simulink model "pwm_deadtime_compensation_model"  (R2023b)
settings: Solver=FixedStepDiscrete  StartTime=0.0  StopTime=deadtime_comp_defaults.simcfg.stop_time  FixedStep=deadtime_comp_defaults.simcfg.Ts_step  RelTol=1e-3
values from neighbouring files (symbols this model uses):
  DeadtimeCompCurrentInvRange_1perA = 12.5    [pwm_deadtime_compensation_interface.sldd]
  DeadtimeCompCurrentZero_A = 0.019999999552965164    [pwm_deadtime_compensation_interface.sldd]
  DeadtimeCompDuty = 0.0099999997764825821    [pwm_deadtime_compensation_interface.sldd]
  DeadtimeCompEnable = 1.0    [pwm_deadtime_compensation_interface.sldd]
  DeadtimeCompPolarity = -1.0    [pwm_deadtime_compensation_interface.sldd]
undefined symbols (not defined in the file or in its folder): deadtime_comp_defaults, deadtime_comp_test
settings Model: DataDictionary=pwm_deadtime_compensation_interface.sldd  Creator=user  LastModifiedBy=user
settings OptimizationCC: DefaultParameterBehavior=Inlined  EnhancedBackFolding=on  PassReuseOutputArgsAs=Individual arguments  OptimizeBlockOrder=speed  DifferentSizesBufferReuse=on  OptimizationCustomize=off  EfficientTunableParamExpr=on
settings DebuggingCC: ParameterTunabilityLossMsg=error
settings HardwareCC: ProdBitPerPointer=32  ProdBitPerSizeT=32  ProdBitPerPtrDiffT=32  ProdLargestAtomicInteger=Long  ProdLargestAtomicFloat=Double  ProdWordSize=32  ProdHWDeviceType=ARM Compatible->ARM Cortex  TargetLargestAtomicInteger=Long  TargetLargestAtomicFloat=Double  TargetIntDivRoundTo=Zero  TargetEndianess=LittleEndian  TargetHWDeviceType=ARM Compatible->ARM Cortex  ProdEqTarget=off
settings SFSimCC: MATLABDynamicMemAlloc=off
settings RTWCC: Description=Embedded Coder  SystemTargetFile=ert.tlc  GenCodeOnly=on  TemplateMakefile=ert_default_tmf  GenerateReport=on
settings CodeAppCC: ForceParamTrailComments=on  IgnoreCustomStorageClasses=off  OperatorAnnotations=on  SimulinkDataObjDesc=on  SFDataObjDesc=on  InsertBlockDesc=on
settings ERTTargetCC: TargetLangStandard=C99 (ISO)  CodeInterfacePackaging=Reusable function  InlinedParameterPlacement=NonHierarchical  ERTCustomFileTemplate=example_file_process.tlc

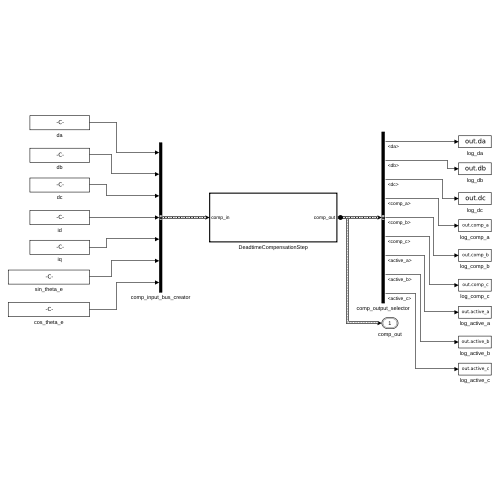
[thumbnail: Simulink's stored preview of the top-level diagram]
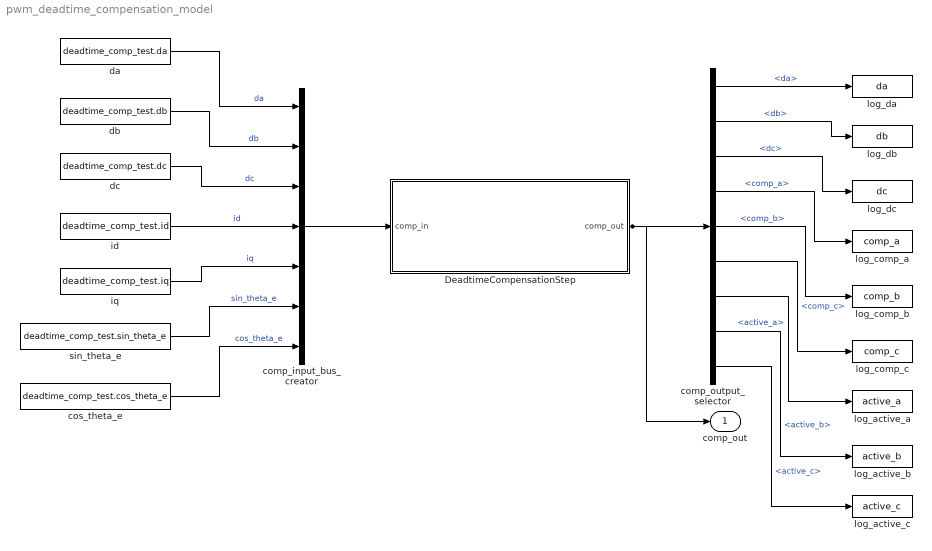
== system pwm_deadtime_compensation_model ==
  DeadtimeCompensationStep : Subsystem  TreatAsAtomicUnit=on  RTWFcnName=DeadtimeCompensationStep  RTWFileName=DeadtimeCompensationStep
      settings: RTWFcnNameOpts=User specified  RTWFileNameOpts=User specified
  comp_input_bus_creator : BusCreator  Inputs=7  OutDataTypeStr=Bus: pwm_deadtime_comp_input_t  NonVirtualBus=on
  comp_output_selector : BusSelector  OutputSignals=da,db,dc,comp_a,comp_b,comp_c,active_a,active_b,active_c
  cos_theta_e : Constant  Value=deadtime_comp_test.cos_theta_e  OutDataTypeStr=T_DeadtimeCompTrig  SampleTime=deadtime_comp_defaults.simcfg.Ts_step
  da : Constant  Value=deadtime_comp_test.da  OutDataTypeStr=T_DeadtimeCompDuty  SampleTime=deadtime_comp_defaults.simcfg.Ts_step
  db : Constant  Value=deadtime_comp_test.db  OutDataTypeStr=T_DeadtimeCompDuty  SampleTime=deadtime_comp_defaults.simcfg.Ts_step
  dc : Constant  Value=deadtime_comp_test.dc  OutDataTypeStr=T_DeadtimeCompDuty  SampleTime=deadtime_comp_defaults.simcfg.Ts_step
  id : Constant  Value=deadtime_comp_test.id  OutDataTypeStr=T_DeadtimeCompCurrent  SampleTime=deadtime_comp_defaults.simcfg.Ts_step
  iq : Constant  Value=deadtime_comp_test.iq  OutDataTypeStr=T_DeadtimeCompCurrent  SampleTime=deadtime_comp_defaults.simcfg.Ts_step
  log_active_a : ToWorkspace  VariableName=active_a  SaveFormat=Structure With Time  SampleTime=-1
  log_active_b : ToWorkspace  VariableName=active_b  SaveFormat=Structure With Time  SampleTime=-1
  log_active_c : ToWorkspace  VariableName=active_c  SaveFormat=Structure With Time  SampleTime=-1
  log_comp_a : ToWorkspace  VariableName=comp_a  SaveFormat=Structure With Time  SampleTime=-1
  log_comp_b : ToWorkspace  VariableName=comp_b  SaveFormat=Structure With Time  SampleTime=-1
  log_comp_c : ToWorkspace  VariableName=comp_c  SaveFormat=Structure With Time  SampleTime=-1
  log_da : ToWorkspace  VariableName=da  SaveFormat=Structure With Time  SampleTime=-1
  log_db : ToWorkspace  VariableName=db  SaveFormat=Structure With Time  SampleTime=-1
  log_dc : ToWorkspace  VariableName=dc  SaveFormat=Structure With Time  SampleTime=-1
  sin_theta_e : Constant  Value=deadtime_comp_test.sin_theta_e  OutDataTypeStr=T_DeadtimeCompTrig  SampleTime=deadtime_comp_defaults.simcfg.Ts_step
  comp_out : Outport  OutDataTypeStr=Bus: pwm_deadtime_comp_output_t  PortDimensions=1
  wires:
  comp_output_selector/7 -> log_active_a/1  "<active_a>"
  comp_output_selector/6 -> log_comp_c/1  "<comp_c>"
  da/1 -> comp_input_bus_creator/1  "da"
  dc/1 -> comp_input_bus_creator/3  "dc"
  db/1 -> comp_input_bus_creator/2  "db"
  DeadtimeCompensationStep/1(comp_out) -> comp_output_selector/1, comp_out/1
  id/1 -> comp_input_bus_creator/4  "id"
  iq/1 -> comp_input_bus_creator/5  "iq"
  sin_theta_e/1 -> comp_input_bus_creator/6  "sin_theta_e"
  comp_output_selector/5 -> log_comp_b/1  "<comp_b>"
  cos_theta_e/1 -> comp_input_bus_creator/7  "cos_theta_e"
  comp_output_selector/8 -> log_active_b/1  "<active_b>"
  comp_input_bus_creator/1 -> DeadtimeCompensationStep/1(comp_in)
  comp_output_selector/9 -> log_active_c/1  "<active_c>"
  comp_output_selector/2 -> log_db/1  "<db>"
  comp_output_selector/3 -> log_dc/1  "<dc>"
  comp_output_selector/1 -> log_da/1  "<da>"
  comp_output_selector/4 -> log_comp_a/1  "<comp_a>"

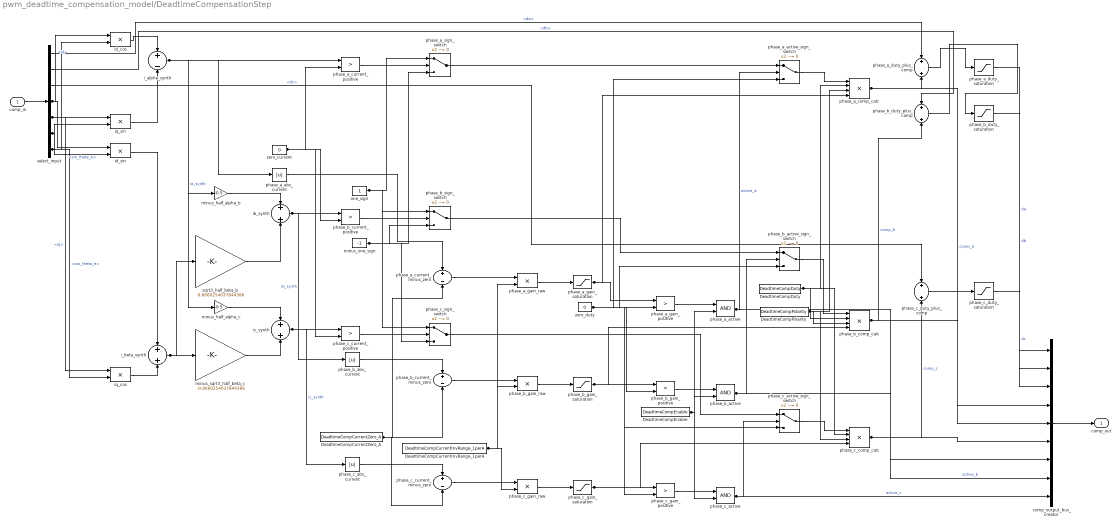
== system pwm_deadtime_compensation_model/DeadtimeCompensationStep ==
  comp_in : Inport  OutDataTypeStr=Bus: pwm_deadtime_comp_input_t  PortDimensions=1  BusOutputAsStruct=on
  DeadtimeCompCurrentInvRange_1perA : Constant  Value=DeadtimeCompCurrentInvRange_1perA  OutDataTypeStr=T_DeadtimeCompDuty  SampleTime=-1
  DeadtimeCompCurrentZero_A : Constant  Value=DeadtimeCompCurrentZero_A  OutDataTypeStr=T_DeadtimeCompCurrent  SampleTime=-1
  DeadtimeCompDuty : Constant  Value=DeadtimeCompDuty  OutDataTypeStr=T_DeadtimeCompDuty  SampleTime=-1
  DeadtimeCompEnable : Constant  Value=DeadtimeCompEnable  OutDataTypeStr=T_DeadtimeCompBool  SampleTime=-1
  DeadtimeCompPolarity : Constant  Value=DeadtimeCompPolarity  OutDataTypeStr=T_DeadtimeCompDuty  SampleTime=-1
  comp_output_bus_creator : BusCreator  Inputs=9  OutDataTypeStr=Bus: pwm_deadtime_comp_output_t  NonVirtualBus=on
  i_alpha_synth : Sum  Inputs=+-  OutDataTypeStr=T_DeadtimeCompCurrent
  i_beta_synth : Sum  OutDataTypeStr=T_DeadtimeCompCurrent
  ib_synth : Sum  OutDataTypeStr=T_DeadtimeCompCurrent
  ic_synth : Sum  OutDataTypeStr=T_DeadtimeCompCurrent
  id_cos : Product  Inputs=**  OutDataTypeStr=T_DeadtimeCompCurrent
  id_sin : Product  Inputs=**  OutDataTypeStr=T_DeadtimeCompCurrent
  iq_cos : Product  Inputs=**  OutDataTypeStr=T_DeadtimeCompCurrent
  iq_sin : Product  Inputs=**  OutDataTypeStr=T_DeadtimeCompCurrent
  minus_half_alpha_b : Gain  Gain=-0.5  OutDataTypeStr=T_DeadtimeCompCurrent
  minus_half_alpha_c : Gain  Gain=-0.5  OutDataTypeStr=T_DeadtimeCompCurrent
  minus_one_sign : Constant  Value=-1  OutDataTypeStr=T_DeadtimeCompDuty  SampleTime=-1
  minus_sqrt3_half_beta_c : Gain  Gain=-0.8660254037844386  OutDataTypeStr=T_DeadtimeCompCurrent
  one_sign : Constant  OutDataTypeStr=T_DeadtimeCompDuty  SampleTime=-1
  phase_a_abs_current : Abs  SaturateOnIntegerOverflow=off
  phase_a_active : Logic  AllPortsSameDT=off  OutDataTypeStr=T_DeadtimeCompBool
  phase_a_active_sign_switch : Switch  Criteria=u2 ~= 0  OutDataTypeStr=T_DeadtimeCompDuty  SaturateOnIntegerOverflow=off  InputSameDT=off
  phase_a_comp_calc : Product  Inputs=****  OutDataTypeStr=T_DeadtimeCompDuty
  phase_a_current_minus_zero : Sum  Inputs=+-  OutDataTypeStr=T_DeadtimeCompCurrent
  phase_a_current_positive : RelationalOperator  Operator=>  OutDataTypeStr=boolean  RndMeth=Simplest  InputSameDT=off
  phase_a_duty_plus_comp : Sum  OutDataTypeStr=T_DeadtimeCompDuty
  phase_a_duty_saturation : Saturate  UpperLimit=1  LowerLimit=0  OutDataTypeStr=T_DeadtimeCompDuty
  phase_a_gain_positive : RelationalOperator  Operator=>  OutDataTypeStr=boolean  RndMeth=Simplest  InputSameDT=off
  phase_a_gain_raw : Product  Inputs=**  OutDataTypeStr=T_DeadtimeCompDuty
  phase_a_gain_saturation : Saturate  UpperLimit=1  LowerLimit=0  OutDataTypeStr=T_DeadtimeCompDuty
  phase_a_sign_switch : Switch  Criteria=u2 ~= 0  OutDataTypeStr=T_DeadtimeCompDuty  SaturateOnIntegerOverflow=off  InputSameDT=off
  phase_b_abs_current : Abs  SaturateOnIntegerOverflow=off
  phase_b_active : Logic  AllPortsSameDT=off  OutDataTypeStr=T_DeadtimeCompBool
  phase_b_active_sign_switch : Switch  Criteria=u2 ~= 0  OutDataTypeStr=T_DeadtimeCompDuty  SaturateOnIntegerOverflow=off  InputSameDT=off
  phase_b_comp_calc : Product  Inputs=****  OutDataTypeStr=T_DeadtimeCompDuty
  phase_b_current_minus_zero : Sum  Inputs=+-  OutDataTypeStr=T_DeadtimeCompCurrent
  phase_b_current_positive : RelationalOperator  Operator=>  OutDataTypeStr=boolean  RndMeth=Simplest  InputSameDT=off
  phase_b_duty_plus_comp : Sum  OutDataTypeStr=T_DeadtimeCompDuty
  phase_b_duty_saturation : Saturate  UpperLimit=1  LowerLimit=0  OutDataTypeStr=T_DeadtimeCompDuty
  phase_b_gain_positive : RelationalOperator  Operator=>  OutDataTypeStr=boolean  RndMeth=Simplest  InputSameDT=off
  phase_b_gain_raw : Product  Inputs=**  OutDataTypeStr=T_DeadtimeCompDuty
  phase_b_gain_saturation : Saturate  UpperLimit=1  LowerLimit=0  OutDataTypeStr=T_DeadtimeCompDuty
  phase_b_sign_switch : Switch  Criteria=u2 ~= 0  OutDataTypeStr=T_DeadtimeCompDuty  SaturateOnIntegerOverflow=off  InputSameDT=off
  phase_c_abs_current : Abs  SaturateOnIntegerOverflow=off
  phase_c_active : Logic  AllPortsSameDT=off  OutDataTypeStr=T_DeadtimeCompBool
  phase_c_active_sign_switch : Switch  Criteria=u2 ~= 0  OutDataTypeStr=T_DeadtimeCompDuty  SaturateOnIntegerOverflow=off  InputSameDT=off
  phase_c_comp_calc : Product  Inputs=****  OutDataTypeStr=T_DeadtimeCompDuty
  phase_c_current_minus_zero : Sum  Inputs=+-  OutDataTypeStr=T_DeadtimeCompCurrent
  phase_c_current_positive : RelationalOperator  Operator=>  OutDataTypeStr=boolean  RndMeth=Simplest  InputSameDT=off
  phase_c_duty_plus_comp : Sum  OutDataTypeStr=T_DeadtimeCompDuty
  phase_c_duty_saturation : Saturate  UpperLimit=1  LowerLimit=0  OutDataTypeStr=T_DeadtimeCompDuty
  phase_c_gain_positive : RelationalOperator  Operator=>  OutDataTypeStr=boolean  RndMeth=Simplest  InputSameDT=off
  phase_c_gain_raw : Product  Inputs=**  OutDataTypeStr=T_DeadtimeCompDuty
  phase_c_gain_saturation : Saturate  UpperLimit=1  LowerLimit=0  OutDataTypeStr=T_DeadtimeCompDuty
  phase_c_sign_switch : Switch  Criteria=u2 ~= 0  OutDataTypeStr=T_DeadtimeCompDuty  SaturateOnIntegerOverflow=off  InputSameDT=off
  select_input : BusSelector  OutputSignals=da,db,dc,id,iq,sin_theta_e,cos_theta_e
  sqrt3_half_beta_b : Gain  Gain=0.8660254037844386  OutDataTypeStr=T_DeadtimeCompCurrent
  zero_current : Constant  Value=0  OutDataTypeStr=T_DeadtimeCompCurrent  SampleTime=-1
  zero_duty : Constant  Value=0  OutDataTypeStr=T_DeadtimeCompDuty  SampleTime=-1
  comp_out : Outport  OutDataTypeStr=Bus: pwm_deadtime_comp_output_t  PortDimensions=1
  wires:
  comp_output_bus_creator/1 -> comp_out/1
  phase_b_duty_saturation/1 -> comp_output_bus_creator/2  "db"
  phase_a_duty_saturation/1 -> comp_output_bus_creator/1  "da"
  phase_b_duty_plus_comp/1 -> phase_b_duty_saturation/1
  phase_a_duty_plus_comp/1 -> phase_a_duty_saturation/1
  DeadtimeCompCurrentZero_A/1 -> phase_a_current_minus_zero/2, phase_b_current_minus_zero/2, phase_c_current_minus_zero/2
  ib_synth/1 -> phase_b_current_positive/1, phase_b_abs_current/1  "ib_synth"
  phase_a_current_positive/1 -> phase_a_sign_switch/2
  phase_c_current_positive/1 -> phase_c_sign_switch/2
  phase_b_current_positive/1 -> phase_b_sign_switch/2
  select_input/2 -> phase_b_duty_plus_comp/1  "<db>"
  minus_half_alpha_c/1 -> ic_synth/1
  sqrt3_half_beta_b/1 -> ib_synth/2
  one_sign/1 -> phase_b_sign_switch/1, phase_a_sign_switch/1, phase_c_sign_switch/1
  phase_a_current_minus_zero/1 -> phase_a_gain_raw/1
  phase_b_gain_positive/1 -> phase_b_active/1
  minus_one_sign/1 -> phase_b_sign_switch/3, phase_c_sign_switch/3, phase_a_sign_switch/3
  phase_c_duty_saturation/1 -> comp_output_bus_creator/3  "dc"
  select_input/5 -> iq_cos/1, iq_sin/1  "<iq>"
  ic_synth/1 -> phase_c_current_positive/1, phase_c_abs_current/1  "ic_synth"
  phase_a_abs_current/1 -> phase_a_current_minus_zero/1
  phase_c_gain_saturation/1 -> phase_c_gain_positive/1, phase_c_comp_calc/4
  i_beta_synth/1 -> minus_sqrt3_half_beta_c/1, sqrt3_half_beta_b/1
  iq_sin/1 -> i_alpha_synth/2
  DeadtimeCompDuty/1 -> phase_b_comp_calc/2, phase_c_comp_calc/2, phase_a_comp_calc/2
  select_input/3 -> phase_c_duty_plus_comp/1  "<dc>"
  phase_b_abs_current/1 -> phase_b_current_minus_zero/1
  DeadtimeCompEnable/1 -> phase_b_active/2, phase_c_active/2, phase_a_active/2
  iq_cos/1 -> i_beta_synth/2
  phase_b_active/1 -> phase_b_active_sign_switch/2, comp_output_bus_creator/8  "active_b"
  phase_c_active/1 -> phase_c_active_sign_switch/2, comp_output_bus_creator/9  "active_c"
  phase_a_comp_calc/1 -> phase_a_duty_plus_comp/2, comp_output_bus_creator/4  "comp_a"
  phase_a_active/1 -> phase_a_active_sign_switch/2, comp_output_bus_creator/7  "active_a"
  i_alpha_synth/1 -> minus_half_alpha_c/1, phase_a_abs_current/1, minus_half_alpha_b/1, phase_a_current_positive/1  "ia_synth"
  select_input/4 -> id_sin/1, id_cos/1  "<id>"
  DeadtimeCompPolarity/1 -> phase_b_comp_calc/3, phase_a_comp_calc/3, phase_c_comp_calc/3
  comp_in/1 -> select_input/1
  phase_c_active_sign_switch/1 -> phase_c_comp_calc/1
  select_input/6 -> id_sin/2, iq_sin/2  "<sin_theta_e>"
  phase_b_current_minus_zero/1 -> phase_b_gain_raw/1
  zero_current/1 -> phase_b_current_positive/2, phase_c_current_positive/2, phase_a_current_positive/2
  select_input/7 -> iq_cos/2, id_cos/2  "<cos_theta_e>"
  id_cos/1 -> i_alpha_synth/1
  id_sin/1 -> i_beta_synth/1
  phase_c_sign_switch/1 -> phase_c_active_sign_switch/1
  phase_c_abs_current/1 -> phase_c_current_minus_zero/1
  phase_a_sign_switch/1 -> phase_a_active_sign_switch/1
  phase_c_comp_calc/1 -> phase_c_duty_plus_comp/2, comp_output_bus_creator/6  "comp_c"
  phase_b_sign_switch/1 -> phase_b_active_sign_switch/1
  phase_a_active_sign_switch/1 -> phase_a_comp_calc/1
  minus_half_alpha_b/1 -> ib_synth/1
  DeadtimeCompCurrentInvRange_1perA/1 -> phase_b_gain_raw/2, phase_c_gain_raw/2, phase_a_gain_raw/2
  phase_c_duty_plus_comp/1 -> phase_c_duty_saturation/1
  phase_c_current_minus_zero/1 -> phase_c_gain_raw/1
  select_input/1 -> phase_a_duty_plus_comp/1  "<da>"
  phase_a_gain_raw/1 -> phase_a_gain_saturation/1
  phase_b_gain_raw/1 -> phase_b_gain_saturation/1
  phase_a_gain_saturation/1 -> phase_a_gain_positive/1, phase_a_comp_calc/4
  phase_c_gain_raw/1 -> phase_c_gain_saturation/1
  zero_duty/1 -> phase_b_gain_positive/2, phase_a_gain_positive/2, phase_a_active_sign_switch/3, phase_c_active_sign_switch/3, phase_c_gain_positive/2, phase_b_active_sign_switch/3
  minus_sqrt3_half_beta_c/1 -> ic_synth/2
  phase_c_gain_positive/1 -> phase_c_active/1
  phase_b_gain_saturation/1 -> phase_b_gain_positive/1, phase_b_comp_calc/4
  phase_a_gain_positive/1 -> phase_a_active/1
  phase_b_active_sign_switch/1 -> phase_b_comp_calc/1
  phase_b_comp_calc/1 -> phase_b_duty_plus_comp/2, comp_output_bus_creator/5  "comp_b"
